simulink model "FOC_PMSM_simulink_block"  (R2018b)
settings: Solver=ode45  StartTime=0.0  StopTime=10.0  RelTol=1e-3  EnableMultiTasking=on
values from neighbouring files (symbols this model uses):
  fs = 5e3    (= 5000)    [Ini_func_for_para_ref_only.m]
  i_maxim_PM = 35    [Ini_func_for_para_ref_only.m]
  Ka_current_d = 170    [Ini_func_for_para_ref_only.m]
  Ka_current_q = 170    [Ini_func_for_para_ref_only.m]
  Ki_current_d = 90*0    (= 0)    [Ini_func_for_para_ref_only.m]
  Ki_current_q = 90*0    (= 0)    [Ini_func_for_para_ref_only.m]
  Ki_speed = 2.2*0    (= 0)    [Ini_func_for_para_ref_only.m]
  Kp_current_d = 3.9    [Ini_func_for_para_ref_only.m]
  Kp_current_q = 3.9*0    (= 0)    [Ini_func_for_para_ref_only.m]
  Kp_speed = 0.13*0    (= 0)    [Ini_func_for_para_ref_only.m]
  lambda_m = 0.123    [Ini_func_for_para_ref_only.m]
  Ld = 2e-3    (= 0.002)    [Ini_func_for_para_ref_only.m]
  Lq = 2e-3    (= 0.002)    [Ini_func_for_para_ref_only.m]
  npp_PM = 4    [Ini_func_for_para_ref_only.m]
  T_PM_limit = 14    [Ini_func_for_para_ref_only.m]
  Td = 1.5*1/5000    (= 0.0003)    [Ini_func_for_para_ref_only.m]
  Udc_max_PM = 650    [Ini_func_for_para_ref_only.m]
  Udc_min_PM = 400    [Ini_func_for_para_ref_only.m]
  Vdq_limit = 300    [Ini_func_for_para_ref_only.m]
undefined symbols (not defined in the file or in its folder): dfilt, DiscIntNeverNeededParam, getIIRFilterDesignOutput
libraries: dspobslib x2, simulink x1
settings Model: Creator=klu  LastModifiedBy=estef
settings DataIOCC: LimitDataPoints=on  SaveFormat=Array
settings OptimizationCC: LifeSpan=inf
settings DebuggingCC: SolverPrmCheckMsg=warning  SFUnexpectedBacktrackingDiag=warning  SFNoUnconditionalDefaultTransitionDiag=warning  SFExecutionAtInitializationDiag=none
settings HardwareCC: ProdBitPerPointer=32  ProdBitPerSizeT=32  ProdBitPerPtrDiffT=32  ProdLargestAtomicFloat=None  ProdIntDivRoundTo=Undefined  ProdEndianess=Unspecified  ProdWordSize=32  ProdHWDeviceType=32-bit Generic
settings ModelReferenceCC: PropagateSignalLabelsOutOfModel=off
settings SFSimCC: SimUseLocalCustomCode=off
settings RTWCC: RTWUseLocalCustomCode=off
settings CodeAppCC: StateflowObjectComments=on
settings GRTTargetCC: TargetLangStandard=C89/C90 (ANSI)  GeneratePreprocessorConditionals=Disable all
settings ConfigComp: CovMetricSettings=dw  CovHtmlReporting=on  CovSaveCumulativeToWorkspaceVar=on  CovSaveSingleToWorkspaceVar=on  CovExternalEMLEnable=off  CovSFcnEnable=off

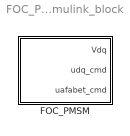
== system FOC_PMSM_simulink_block ==
  FOC_PMSM : Subsystem
      mask Display: disp('FOC PMSM')

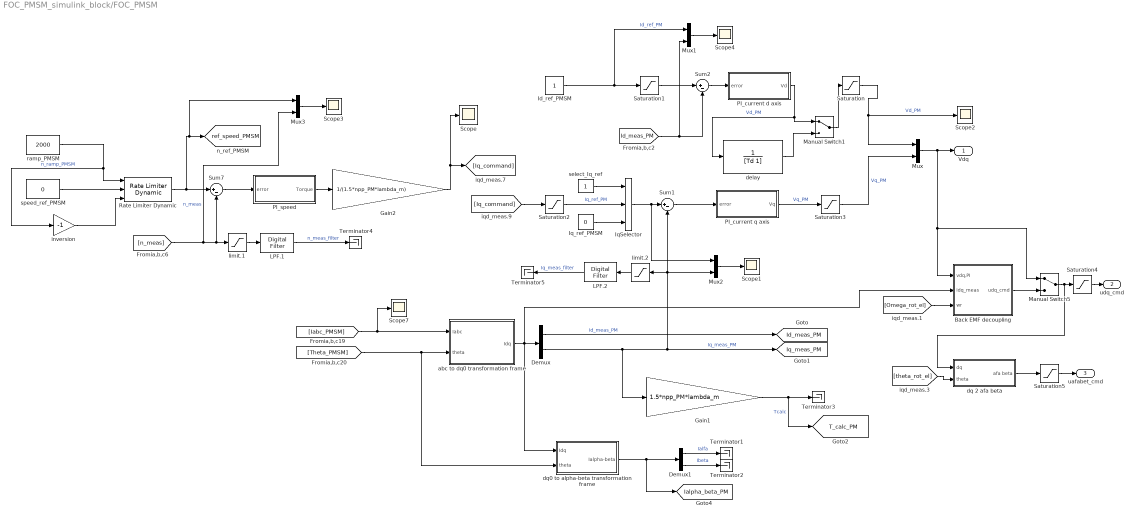
== system FOC_PMSM_simulink_block/FOC_PMSM ==
  Back EMF decoupling : Subsystem
  Demux : Demux  Outputs=2
  Demux1 : Demux  Outputs=2
  Gain1 : Gain  Gain=1.5*npp_PM*lambda_m
  Gain2 : Gain  Gain=1/(1.5*npp_PM*lambda_m)
  Id_ref_PMSM : Constant
  IqSelector : MultiPortSwitch  Inputs=2  SaturateOnIntegerOverflow=on  InputSameDT=on
  Iq_ref_PMSM : Constant  Value=0
  LPF.1 : dspobslib/Digital Filter  TypePopup=IIR (poles & zeros)  IIRFiltStruct=Direct form II transposed  AllPoleFiltStruct=Direct form  FIRFiltStruct=Direct form  CoeffSource=Specify via dialog  NumCoeffs=getIIRFilterDesignOutput('Butterworth','Lowpass',2,2,20,0.5/(fs/2),0.6,1)  DenCoeffs=getIIRFilterDesignOutput('Butterworth','Lowpass',2,2,20,0.5/(fs/2),0.6,2)  BiQuadCoeffs=[1 0.3 0.4 1 0.1 0.2]  LatticeCoeffs=[0.2 0.4]  denIgnore=on  FiltPerSampPopup=One filter per frame  IC=0  ICnum=0  ICden=0  roundingMode=Floor  overflowMode=off  ScaleValues=1  scaleValueFracLength=14  stageInFracLength=15  stageOutFracLength=15  FilterSource=Specify via dialog  dfiltObjectName=dfilt.dffir([1 2 1])  InputProcessing=Inherited (this choice will be removed - see release notes)
      settings: SourceProductName=DSP System Toolbox  SourceProductBaseCode=DS
  LPF.2 : dspobslib/Digital Filter  TypePopup=IIR (poles & zeros)  IIRFiltStruct=Direct form II transposed  AllPoleFiltStruct=Direct form  FIRFiltStruct=Direct form  CoeffSource=Specify via dialog  NumCoeffs=getIIRFilterDesignOutput('Butterworth','Lowpass',2,2,20,0.5/(fs/2),0.6,1)  DenCoeffs=getIIRFilterDesignOutput('Butterworth','Lowpass',2,2,20,0.5/(fs/2),0.6,2)  BiQuadCoeffs=[1 0.3 0.4 1 0.1 0.2]  LatticeCoeffs=[0.2 0.4]  denIgnore=on  FiltPerSampPopup=One filter per frame  IC=0  ICnum=0  ICden=0  roundingMode=Floor  overflowMode=off  ScaleValues=1  scaleValueFracLength=14  stageInFracLength=15  stageOutFracLength=15  FilterSource=Specify via dialog  dfiltObjectName=dfilt.dffir([1 2 1])  InputProcessing=Inherited (this choice will be removed - see release notes)
      settings: SourceProductName=DSP System Toolbox  SourceProductBaseCode=DS
  Manual Switch1 : ManualSwitch
  Manual Switch5 : ManualSwitch
  Mux{,1..3} (4 alike) : Mux  Inputs=2
  PI_current d axis : Subsystem
  PI_current q axis : Subsystem
  PI_speed : Subsystem
  Rate Limiter Dynamic : simulink/Discontinuities/Rate Limiter Dynamic
      settings: SourceProductName=Simulink
  Saturation{,3..5} (4 alike) : Saturate  UpperLimit=Udc_max_PM  LowerLimit=Udc_min_PM
  Saturation1 : Saturate  UpperLimit=i_maxim_PM  LowerLimit=-i_maxim_PM
  Saturation2 : Saturate  UpperLimit=i_maxim_PM  LowerLimit=-i_maxim_PM
  Scope{,1..4,7} (6 alike) : Scope
  Sum1 : Sum  Inputs=|+-
  Sum2 : Sum  Inputs=|+-
  Sum7 : Sum  Inputs=|+-
  Terminator{1..5} (5 alike) : Terminator
  abc to dq0 transformation frame : Subsystem
  "delay " : TransferFcn  Denominator=[Td 1]
  dq 2 afa beta : Subsystem
  dq0 to alpha-beta transformation frame : Subsystem
  inversion : Gain  Gain=-1
  limit.1 : Saturate  UpperLimit=5000  LowerLimit=-5000
  limit.2 : Saturate  UpperLimit=5000  LowerLimit=-5000
  ramp_PMSM : Constant  Value=2000  SampleTime=-1
  select_Iq_ref : Constant  SampleTime=-1
  speed_ref_PMSM : Constant  Value=0  SampleTime=-1
  Vdq : Outport
  udq_cmd : Outport  Port=2
  uafabet_cmd : Outport  Port=3
  tag scope: Ialpha_beta_PM=global, Id_meas_PM=global, Iq_meas_PM=global, T_calc_PM=global, ref_speed_PMSM=global
  wires:
  [n_meas] -> Mux3/2, limit.1/1, Sum7/2  "n_meas"
  [Theta_PMSM] -> dq0 to alpha-beta transformation frame/2(theta), abc to dq0 transformation frame/2(theta)
  Demux/1 -> [Id_meas_PM]  "Id_meas_PM"
  Sum1/1 -> PI_current q axis/1(error)
  dq0 to alpha-beta transformation frame/1(Ialpha-beta) -> Demux1/1, [Ialpha_beta_PM]
  Demux1/1 -> Terminator1/1  "Ialfa"
  Demux1/2 -> Terminator2/1  "Ibeta"
  abc to dq0 transformation frame/1(Idq) -> Back EMF decoupling/2(idq_meas), Demux/1, dq0 to alpha-beta transformation frame/1(Idq)
  Gain1/1 -> [T_calc_PM], Terminator3/1  "Tcalc"
  Demux/2 -> [Iq_meas_PM], Mux2/2, Sum1/2, limit.2/1, Gain1/1  "Iq_meas_PM"
  [Iabc_PMSM] -> Scope7/1, abc to dq0 transformation frame/1(Iabc)
  ramp_PMSM/1 -> Rate Limiter Dynamic/1, inversion/1  "n_ramp_PMSM"
  inversion/1 -> Rate Limiter Dynamic/3
  Rate Limiter Dynamic/1 -> Sum7/1, Mux3/1, [ref_speed_PMSM]
  Saturation2/1 -> IqSelector/2  "Iq_ref_PM"
  IqSelector/1 -> Mux2/1, Sum1/1
  select_Iq_ref/1 -> IqSelector/1
  Iq_ref_PMSM/1 -> IqSelector/3
  speed_ref_PMSM/1 -> Rate Limiter Dynamic/2
  limit.1/1 -> LPF.1/1
  LPF.1/1 -> Terminator4/1  "n_meas_filter"
  limit.2/1 -> LPF.2/1
  LPF.2/1 -> Terminator5/1  "Iq_meas_filter"
  Saturation/1 -> Scope2/1, Mux/1  "Vd_PM"
  Id_ref_PMSM/1 -> Mux1/1, Saturation1/1  "Id_ref_PM"
  Saturation1/1 -> Sum2/1
  [Id_meas_PM] -> Mux1/2, Sum2/2
  Sum2/1 -> PI_current d axis/1(error)
  [Iq_command] -> Saturation2/1
  PI_current q axis/1(Vq) -> Saturation3/1  "Vq_PM"
  Mux/1 -> Manual Switch5/1, Back EMF decoupling/1(vdq,PI), Vdq/1
  Saturation3/1 -> Mux/2  "Vq_PM"
  Sum7/1 -> PI_speed/1(error)
  PI_speed/1(Torque) -> Gain2/1
  Gain2/1 -> Scope/1, [Iq_command]
  Mux1/1 -> Scope4/1
  Mux2/1 -> Scope1/1
  Mux3/1 -> Scope3/1
  Back EMF decoupling/1(udq_cmd) -> Manual Switch5/2
  Saturation4/1 -> udq_cmd/1
  Manual Switch5/1 -> dq 2 afa beta/1(dq), Saturation4/1
  Saturation5/1 -> uafabet_cmd/1
  dq 2 afa beta/1(afa beta) -> Saturation5/1
  [theta_rot_el] -> dq 2 afa beta/2(theta)
  [Omega_rot_el] -> Back EMF decoupling/3(wr)
  PI_current d axis/1(Vd) -> "delay "/1, Manual Switch1/1  "Vd_PM"
  Manual Switch1/1 -> Saturation/1
  "delay "/1 -> Manual Switch1/2

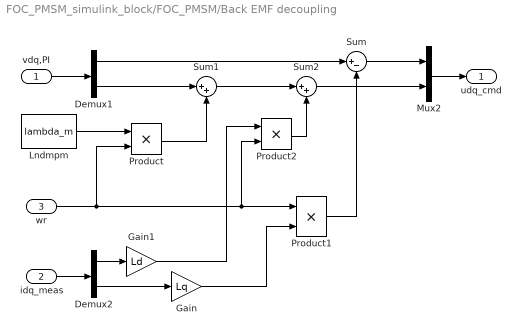
== system FOC_PMSM_simulink_block/FOC_PMSM/Back EMF decoupling ==
  vdq,PI : Inport
  idq_meas : Inport  Port=2
  wr : Inport  Port=3
  Demux1 : Demux  Outputs=2
  Demux2 : Demux  Outputs=2
  Gain : Gain  Gain=Lq
  Gain1 : Gain  Gain=Ld
  Lndmpm : Constant  Value=lambda_m
  Mux2 : Mux  Inputs=2
  Product : Product  RndMeth=Zero
  Product1 : Product  RndMeth=Zero
  Product2 : Product  RndMeth=Zero
  Sum : Sum  Inputs=|+-
  Sum1 : Sum  Inputs=|++
  Sum2 : Sum  Inputs=|++
  udq_cmd : Outport
  wires:
  Mux2/1 -> udq_cmd/1
  vdq,PI/1 -> Demux1/1
  Demux1/1 -> Sum/1
  Sum/1 -> Mux2/1
  Demux1/2 -> Sum1/1
  idq_meas/1 -> Demux2/1
  wr/1 -> Product/2, Product1/1, Product2/2
  Product1/1 -> Sum/2
  Gain/1 -> Product1/2
  Demux2/2 -> Gain/1
  Lndmpm/1 -> Product/1
  Product/1 -> Sum1/2
  Sum1/1 -> Sum2/1
  Demux2/1 -> Gain1/1
  Gain1/1 -> Product2/1
  Product2/1 -> Sum2/2
  Sum2/1 -> Mux2/2

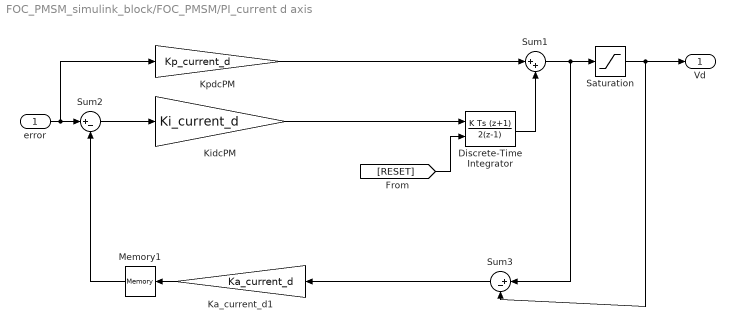
== system FOC_PMSM_simulink_block/FOC_PMSM/PI_current d axis ==
  error : Inport
  Discrete-Time Integrator : DiscreteIntegrator  IntegratorMethod=Integration: Trapezoidal  ExternalReset=level  SampleTime=-1  ICPrevOutput=DiscIntNeverNeededParam  ICPrevScaledInput=DiscIntNeverNeededParam
  Ka_current_d1 : Gain  Gain=Ka_current_d
  KidcPM : Gain  Gain=Ki_current_d
  KpdcPM : Gain  Gain=Kp_current_d
  Memory1 : Memory  InheritSampleTime=on
  Saturation : Saturate  UpperLimit=Vdq_limit  LowerLimit=-Vdq_limit
  Sum1 : Sum  Inputs=|++
  Sum2 : Sum  Inputs=|+-
  Sum3 : Sum  Inputs=|+-
  Vd : Outport
  wires:
  error/1 -> KpdcPM/1, Sum2/1
  KidcPM/1 -> Discrete-Time Integrator/1
  KpdcPM/1 -> Sum1/1
  Discrete-Time Integrator/1 -> Sum1/2
  Sum1/1 -> Saturation/1, Sum3/1
  Saturation/1 -> Vd/1, Sum3/2
  [RESET] -> Discrete-Time Integrator/2
  Ka_current_d1/1 -> Memory1/1
  Sum3/1 -> Ka_current_d1/1
  Memory1/1 -> Sum2/2
  Sum2/1 -> KidcPM/1

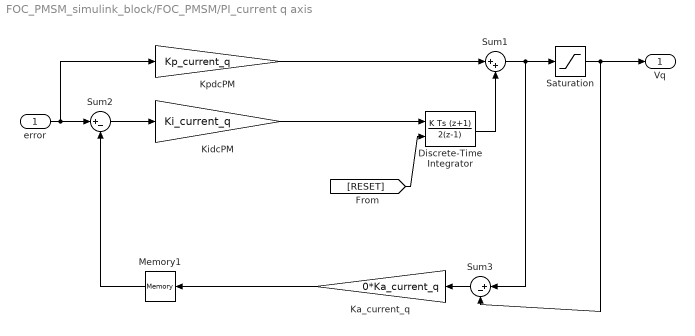
== system FOC_PMSM_simulink_block/FOC_PMSM/PI_current q axis ==
  error : Inport
  Discrete-Time Integrator : DiscreteIntegrator  IntegratorMethod=Integration: Trapezoidal  ExternalReset=level  SampleTime=-1  ICPrevOutput=DiscIntNeverNeededParam  ICPrevScaledInput=DiscIntNeverNeededParam
  Ka_current_q : Gain  Gain=0*Ka_current_q
  KidcPM : Gain  Gain=Ki_current_q
  KpdcPM : Gain  Gain=Kp_current_q
  Memory1 : Memory  InheritSampleTime=on
  Saturation : Saturate  UpperLimit=Vdq_limit  LowerLimit=-Vdq_limit
  Sum1 : Sum  Inputs=|++
  Sum2 : Sum  Inputs=|+-
  Sum3 : Sum  Inputs=|+-
  Vq : Outport
  wires:
  [RESET] -> Discrete-Time Integrator/2
  Saturation/1 -> Vq/1, Sum3/2
  Sum1/1 -> Saturation/1, Sum3/1
  Discrete-Time Integrator/1 -> Sum1/2
  KpdcPM/1 -> Sum1/1
  KidcPM/1 -> Discrete-Time Integrator/1
  error/1 -> KpdcPM/1, Sum2/1
  Ka_current_q/1 -> Memory1/1
  Sum3/1 -> Ka_current_q/1
  Sum2/1 -> KidcPM/1
  Memory1/1 -> Sum2/2

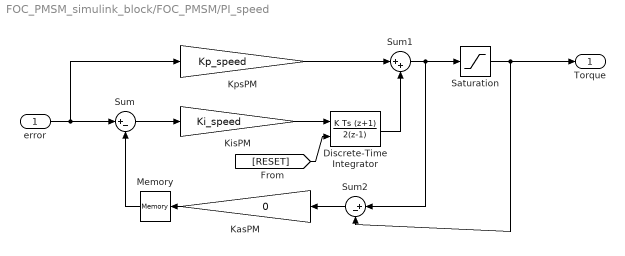
== system FOC_PMSM_simulink_block/FOC_PMSM/PI_speed ==
  error : Inport
  Discrete-Time Integrator : DiscreteIntegrator  IntegratorMethod=Integration: Trapezoidal  ExternalReset=level  SampleTime=-1  ICPrevOutput=DiscIntNeverNeededParam  ICPrevScaledInput=DiscIntNeverNeededParam
  KasPM : Gain  Gain=0
  KisPM : Gain  Gain=Ki_speed
  KpsPM : Gain  Gain=Kp_speed
  Memory : Memory  InheritSampleTime=on
  Saturation : Saturate  UpperLimit=T_PM_limit  LowerLimit=-T_PM_limit
  Sum : Sum  Inputs=|+-
  Sum1 : Sum  Inputs=|++
  Sum2 : Sum  Inputs=|+-
  Torque : Outport
  wires:
  error/1 -> KpsPM/1, Sum/1
  Sum/1 -> KisPM/1
  KisPM/1 -> Discrete-Time Integrator/1
  KpsPM/1 -> Sum1/1
  Discrete-Time Integrator/1 -> Sum1/2
  KasPM/1 -> Memory/1
  Sum2/1 -> KasPM/1
  Sum1/1 -> Sum2/1, Saturation/1
  Saturation/1 -> Sum2/2, Torque/1
  [RESET] -> Discrete-Time Integrator/2
  Memory/1 -> Sum/2

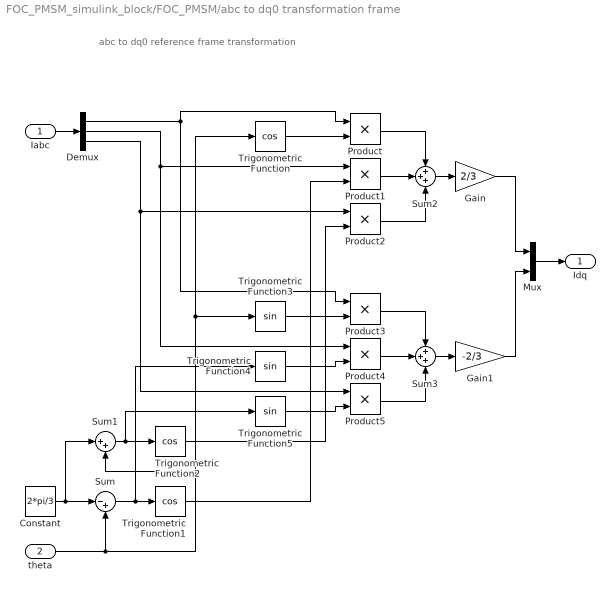
== system FOC_PMSM_simulink_block/FOC_PMSM/abc to dq0 transformation frame ==
  note: abc to dq0 reference frame transformation
  Iabc : Inport
  theta : Inport  Port=2
  Constant : Constant  Value=2*pi/3
  Demux : Demux  Outputs=3
  Gain : Gain  Gain=2/3
  Gain1 : Gain  Gain=-2/3
  Mux : Mux  Inputs=2
  Product{,1..5} (6 alike) : Product  RndMeth=Zero
  Sum : Sum  Inputs=|-+
  Sum1 : Sum  Inputs=|++
  Sum2 : Sum  Inputs=+++
  Sum3 : Sum  Inputs=+++
  Trigonometric Function : Trigonometry  Operator=cos
  Trigonometric Function1 : Trigonometry  Operator=cos
  Trigonometric Function2 : Trigonometry  Operator=cos
  Trigonometric Function3 : Trigonometry
  Trigonometric Function4 : Trigonometry
  Trigonometric Function5 : Trigonometry
  Idq : Outport
  wires:
  Iabc/1 -> Demux/1
  Demux/1 -> Product/1, Product3/1
  Trigonometric Function/1 -> Product/2
  theta/1 -> Sum/2, Sum1/2, Trigonometric Function/1, Trigonometric Function3/1
  Constant/1 -> Sum/1, Sum1/1
  Sum/1 -> Trigonometric Function1/1, Trigonometric Function4/1
  Demux/2 -> Product1/1, Product4/1
  Trigonometric Function1/1 -> Product1/2
  Sum1/1 -> Trigonometric Function2/1, Trigonometric Function5/1
  Trigonometric Function2/1 -> Product2/2
  Demux/3 -> Product2/1, Product5/1
  Product1/1 -> Sum2/2
  Product/1 -> Sum2/1
  Product2/1 -> Sum2/3
  Product4/1 -> Sum3/2
  Product3/1 -> Sum3/1
  Product5/1 -> Sum3/3
  Trigonometric Function3/1 -> Product3/2
  Trigonometric Function5/1 -> Product5/2
  Trigonometric Function4/1 -> Product4/2
  Sum2/1 -> Gain/1
  Sum3/1 -> Gain1/1
  Gain/1 -> Mux/1
  Gain1/1 -> Mux/2
  Mux/1 -> Idq/1

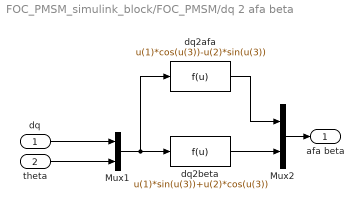
== system FOC_PMSM_simulink_block/FOC_PMSM/dq 2 afa beta ==
  dq : Inport
  theta : Inport  Port=2
  Mux1 : Mux  Inputs=2
  Mux2 : Mux  Inputs=2
  dq2afa : Fcn  Expr=u(1)*cos(u(3))-u(2)*sin(u(3))
  dq2beta : Fcn  Expr=u(1)*sin(u(3))+u(2)*cos(u(3))
  afa beta : Outport
  wires:
  Mux2/1 -> afa beta/1
  dq2beta/1 -> Mux2/2
  dq2afa/1 -> Mux2/1
  Mux1/1 -> dq2afa/1, dq2beta/1
  theta/1 -> Mux1/2
  dq/1 -> Mux1/1

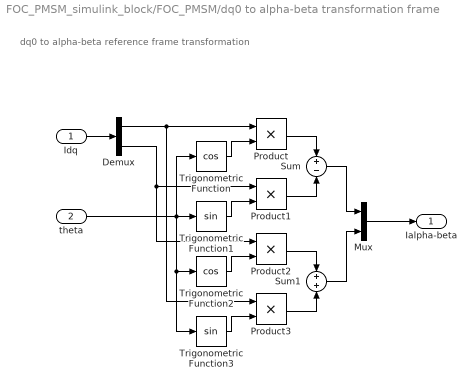
== system FOC_PMSM_simulink_block/FOC_PMSM/dq0 to alpha-beta transformation frame ==
  note: dq0 to alpha-beta reference frame transformation
  Idq : Inport
  theta : Inport  Port=2
  Demux : Demux  Outputs=2
  Mux : Mux  Inputs=2
  Product{,1..3} (4 alike) : Product  RndMeth=Zero
  Sum : Sum  Inputs=+|-
  Sum1 : Sum  Inputs=+|+
  Trigonometric Function : Trigonometry  Operator=cos
  Trigonometric Function1 : Trigonometry
  Trigonometric Function2 : Trigonometry  Operator=cos
  Trigonometric Function3 : Trigonometry
  Ialpha-beta : Outport
  wires:
  Idq/1 -> Demux/1
  theta/1 -> Trigonometric Function/1, Trigonometric Function1/1, Trigonometric Function2/1, Trigonometric Function3/1
  Demux/1 -> Product/1, Product3/1
  Trigonometric Function/1 -> Product/2
  Trigonometric Function1/1 -> Product1/2
  Demux/2 -> Product1/1, Product2/1
  Product/1 -> Sum/1
  Product1/1 -> Sum/2
  Sum/1 -> Mux/1
  Mux/1 -> Ialpha-beta/1
  Trigonometric Function2/1 -> Product2/2
  Trigonometric Function3/1 -> Product3/2
  Product2/1 -> Sum1/1
  Product3/1 -> Sum1/2
  Sum1/1 -> Mux/2
